simulink model "PARTEBSIMULINK"  (R2015a)
settings: Solver=ode45  StartTime=0.0  StopTime=70  RelTol=1e-3
settings Model: Creator=Bruna  LastModifiedBy=WELLITON LEAL (W)
settings DataIOCC: SignalLoggingSaveFormat=ModelDataLogs
settings OptimizationCC: ExpressionDepthLimit=2147483647
settings DebuggingCC: UnderspecifiedInitializationDetection=Classic  MergeDetectMultiDrivingBlocksExec=none  SolverPrmCheckMsg=warning  FcnCallInpInsideContextMsg=UseLocalSettings  StateNameClashWarn=warning
settings GRTTargetCC: CombineOutputUpdateFcns=off  GRTInterface=on

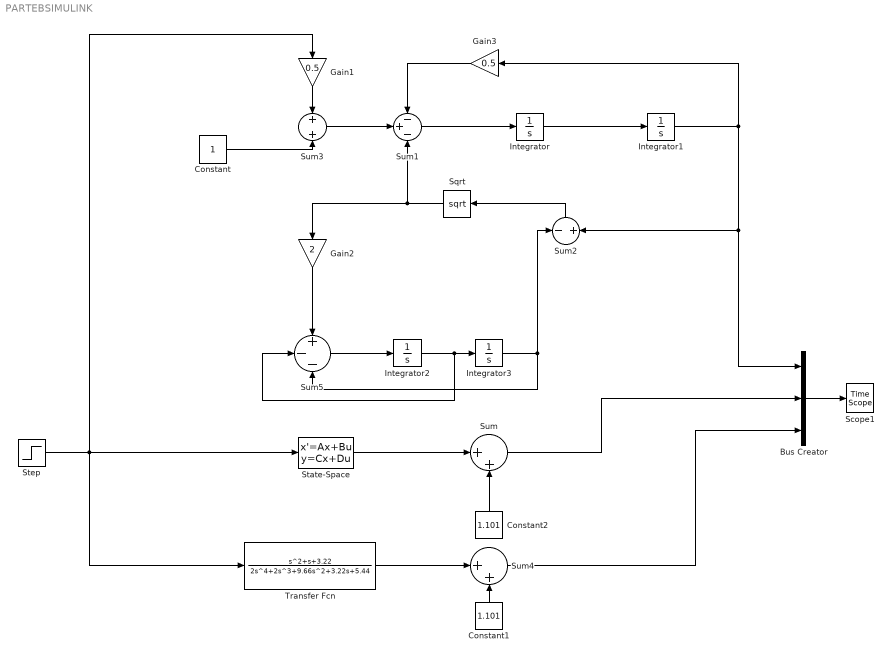
== system PARTEBSIMULINK ==
  Bus Creator : BusCreator  Inputs=3
  Constant : Constant
  Constant1 : Constant  Value=1.101
  Constant2 : Constant  Value=1.101
  Gain1 : Gain  Gain=0.5
  Gain2 : Gain  Gain=2
  Gain3 : Gain  Gain=0.5
  Integrator{,1..3} (4 alike) : Integrator
  Scope1 : TimeScope
  Sqrt : Sqrt  SaturateOnIntegerOverflow=on
  State-Space : StateSpace  A=[0 1 0 0; 3.22 1 -2.22 0; 0 0 0 1; 1.11 0 -1.61 0]  B=[0; 0; 0; 0.5]  C=[0 0 1 0]  D=[0]  X0=0
  Step : Step  Time=120  After=0.1  SampleTime=0
  Sum : Sum  Inputs=|++
  Sum1 : Sum  Inputs=-+-
  Sum2 : Sum  Inputs=-+
  Sum3 : Sum
  Sum4 : Sum  Inputs=|++
  Sum5 : Sum  Inputs=+--
  Transfer Fcn : TransferFcn  Numerator=[1 1 3.22]  Denominator=[2 2 9.66 3.22 5.44]
  wires:
  Step/1 -> Transfer Fcn/1, Gain1/1, State-Space/1
  State-Space/1 -> Sum/1
  Transfer Fcn/1 -> Sum4/1
  Constant1/1 -> Sum4/2
  Constant2/1 -> Sum/2
  Sum4/1 -> Bus Creator/3
  Sum/1 -> Bus Creator/2
  Bus Creator/1 -> Scope1/1
  Integrator/1 -> Integrator1/1
  Sum1/1 -> Integrator/1
  Gain1/1 -> Sum3/1
  Gain3/1 -> Sum1/1
  Integrator1/1 -> Sum2/2, Bus Creator/1, Gain3/1
  Sum2/1 -> Sqrt/1
  Gain2/1 -> Sum5/1
  Integrator2/1 -> Integrator3/1, Sum5/2
  Integrator3/1 -> Sum2/1, Sum5/3
  Sum5/1 -> Integrator2/1
  Sum3/1 -> Sum1/2
  Sqrt/1 -> Sum1/3, Gain2/1
  Constant/1 -> Sum3/2
